simulink library "mbed_lib"  (Simulink 8.3)
settings: Solver=ode45  SolverMode=SingleTasking  StartTime=0.0  StopTime=10.0  RelTol=1e-3
settings Model: Creator=syoon  LastModifiedBy=axel

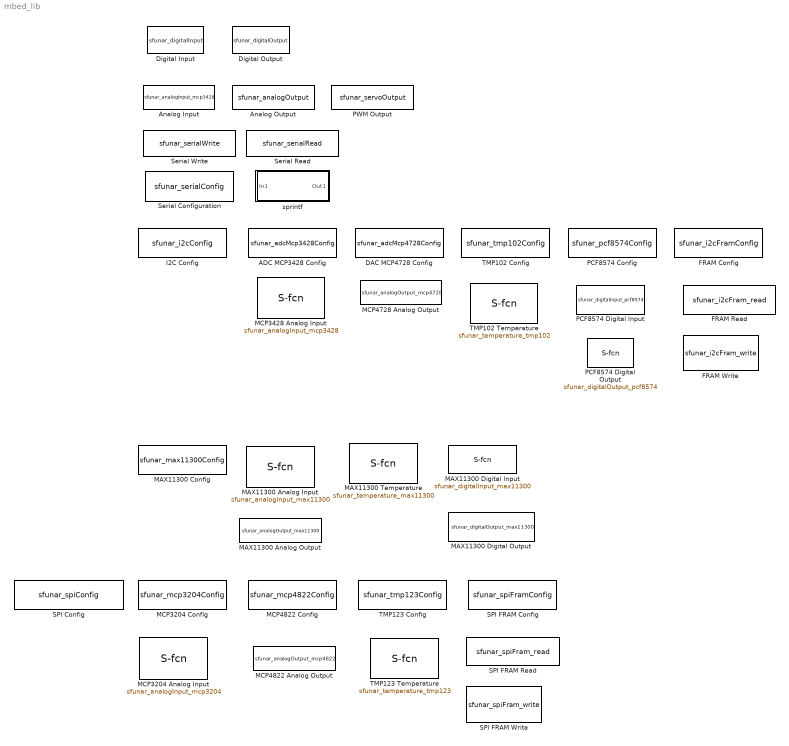
== system mbed_lib ==
  ADC MCP3428 Config : S-Function  Priority=1  AncestorBlock=mbed_lib/I2C Config  FunctionName=sfunar_adcMcp3428Config  Parameters=uint8(SParameter1)  EnableBusSupport=off  mask(MCP3428 Configuration){SParameter1=0}
      mask prompts: SParameter1 "Device Sub Address"
      mask help:
      | This blocks sets up the MCP3428 on the I2C board. You must have one of these blocks in any model that ues this device.
      |
      | The sub-address must match the pin configuration on the board. See the board documentation for details.
      mask Display: disp(['Sub-Address: ' num2str(SParameter1) ]);
  Analog Input : S-Function  FunctionName=sfunar_analogInput_mcp3428  Parameters=uint8(SParameter1), SampleTime  EnableBusSupport=off  mask(Arduino Analog Input){SParameter2=A, SParameter1=0, SampleTime=-1}
      mask prompts: SParameter2 "Port Name:"; SParameter1 "Pin Number (1-16):"; SampleTime "Sample time (-1 for inherited):"
      mask help:
      | Reads the analog voltage input from the specified pin on the Arduino board.
      |
      | The range of input on the pin is between 0 and 5 Volts corresponding to a block output of 0 to 1023.
      mask Help:
      | <p>This block calls the analogRead() function from the Arduino language library.
      | <p>For more information see: <a href="http://arduino.cc/en/Reference/AnalogRead">Arduino - AnalogRead</a>
      mask TypeOptions SParameter2: A | B | C | D | E | F
      mask Display:
      | plot([0:0.05:0.5],0.3*sin(4*pi*[0.5:0.05:1])+0.5)
      | port_label('output',1,['Pin ', SParameter2+64, '.', num2str(SParameter1)]);
  Analog Output : S-Function  FunctionName=sfunar_analogOutput  Parameters=uint8(SParameter1), SampleTime, uint8(SParameter2)  EnableBusSupport=off  mask(Arduino Analog Output){SParameter2=A, SampleTime=-1, SParameter1=0}
      mask prompts: SParameter2 "Port Name:"; SampleTime "Sample time (-1 for inherited):"; SParameter1 "Pin Number (1-16):"
      mask help:
      | Approximates an analog output on the specified pin on the Arduino board using a PWM signal with a frequency of ~490 Hz.
      |
      | The input to this block is an integer between 0 and 255 corresponding to 0 to 5V.
      mask Help:
      | <p>This block calls the analogWrite() function from the Arduino language library.
      | <p>For more information see: <a href="http://arduino.cc/en/Reference/AnalogWrite">Arduino - AnalogWrite</a>
      mask TypeOptions SParameter2: A | B | C | D | E | F
      mask Display:
      | plot([0.5:0.05:1],0.3*sin(4*pi*[0.5:0.05:1])+0.5)
      | port_label('input',1,['Pin ', SParameter2+64, '.', num2str(SParameter1)]);
  DAC MCP4728 Config : S-Function  Priority=1  FunctionName=sfunar_adcMcp4728Config  Parameters=uint8(SParameter1)  EnableBusSupport=off  mask(MCP4728 Configuration){SParameter1=0}
      mask prompts: SParameter1 "Device Sub Address"
      mask help:
      | This blocks sets up the MCP4728 on the I2C board. You must have one of these blocks in any model that ues this device.
      |
      | The sub-address must match the pin configuration on the board. See the board documentation for details.
      mask Display: disp(['Sub-Address: ' num2str(SParameter1) ]);
  Digital Input : S-Function  FunctionName=sfunar_digitalInput  Parameters=uint8(SParameter1), SampleTime, uint8(SParameter2), uint8(SParameter3)  EnableBusSupport=off  mask(Arduino Digital Input){SParameter2=A, SParameter1=0, SParameter3=INPUT, SampleTime=-1}
      mask prompts: SParameter2 "Port Name"; SParameter1 "Pin Number (1-16):"; SParameter3 "Input Mode"; SampleTime "Sample time (-1 for inherited):"
      mask help:
      | Reads the digital value from the specified pin on the Arduino board.
      |
      | It outputs 1 for high and 0 for low.
      mask Help:
      | <p>This block calls the digitalRead() function from the Arduino language library.
      | <p>For more information see: <a href="http://arduino.cc/en/Reference/DigitalRead">Arduino - DigitalRead</a>
      mask TypeOptions SParameter2: A | B | C | D | E | F
      mask TypeOptions SParameter3: INPUT | INPUT_PULLUP | INPUT_PULLDOWN
      mask Display:
      | plot([0 0.15 0.15 0.35 0.35 0.5],[0.3 0.3 0.7 0.7 0.3 0.3])
      | port_label('output',1,['Pin ', SParameter2+64, '.', num2str(SParameter1)]);
  Digital Output : S-Function  FunctionName=sfunar_digitalOutput  Parameters=uint8(SParameter1), SampleTime, uint8(SParameter2), uint8(SParameter3)  EnableBusSupport=off  mask(Arduino Digital Output){SParameter2=D, SParameter1=12, SParameter3=OUTPUT, SampleTime=-1}
      mask prompts: SParameter2 "Port Name:"; SParameter1 "Pin Number(1~16):"; SParameter3 "Output Mode"; SampleTime "Sample time (-1 for inherited):"
      mask help:
      | Sends the digital value to the specified port.pin on the Arduino board.
      | The pin can be configured as push-pull (pp) or open drain output (od).
      |
      | An input of 1 sets the pin high and 0 sets the pin low.
      mask Help:
      | <p>This block calls the digitalWrite() function from the Arduino language library.
      | <p>For init the pinmode function ist called
      | <p>For more information see: <a href="http://arduino.cc/en/Reference/DigitalWrite">Arduino - DigitalWrite</a>
      mask TypeOptions SParameter2: A | B | C | D | E | F
      mask TypeOptions SParameter3: OUTPUT | OUTPUT_OPENDRAIN
      mask Display:
      | plot([0.5 0.65 0.65 0.85 0.85 1],[0.3 0.3 0.7 0.7 0.3 0.3])
      | port_label('input',1,['Pin ', SParameter2+64, '.', num2str(SParameter1)]);
  FRAM Config : S-Function  Priority=1  FunctionName=sfunar_i2cFramConfig  EnableBusSupport=off  mask(I2C Fram Config){}
  FRAM Read : S-Function  FunctionName=sfunar_i2cFram_read  Parameters=uint8(SParameter1-1), SampleTime, boolean(errEn)  EnableBusSupport=off  mask(Fram Read){SampleTime=-1, SParameter1=on startup, errEn=on}
      mask prompts: SampleTime "Sample time (-1 for inherited):"; SParameter1 "Read condition"; errEn "Enable error output port"
      mask help: Reads one byte from the FRAM.
      mask TypeOptions SParameter1: on startup | on each step
      mask Display:
      | port_label('input', 1, 'Page Address');
      | port_label('input', 2, 'Word Address');
      | 
      | port_label('output',1,'Value');
      | if errEn
      | port_label('output',2,'Error');
      | end
  FRAM Write : S-Function  FunctionName=sfunar_i2cFram_write  Parameters=uint8(SParameter1-1), SampleTime, boolean(errEn)  EnableBusSupport=off  mask(FRAM Write){SampleTime=-1, SParameter1=on startup, errEn=on}
      mask prompts: SampleTime "Sample time (-1 for inherited):"; SParameter1 "Write condition"; errEn "Enable error output port"
      mask help: Writes one byte to the FRAM
      mask TypeOptions SParameter1: on startup | on each step
      mask Display:
      | port_label('input', 1, 'Page Address');
      | port_label('input', 2, 'Word Address');
      | port_label('input', 3, 'Data');
      | 
      | if errEn
      | port_label('output',1,'Error');
      | end
  I2C Config : S-Function  Priority=0  AncestorBlock=mbed_lib/Serial Configuration  FunctionName=sfunar_i2cConfig  Parameters=uint8(0), uint8(SParameter2), uint8(SParameter3), uint8(SParameter4), uint8(SParameter5), SParameter6  EnableBusSupport=off  mask(I2C Configuration){SParameter6=100000, SParameter2=B, SParameter3=9, SParameter4=B, SParameter5=8}
      mask prompts: SParameter6 "Bus frequency: [Hz]"; SParameter2 "Port Name (SDA)"; SParameter3 "Pin Number (1-16):"; SParameter4 "Port Name (SCL)"; SParameter5 "Pin Number (1-16):"
      mask help: This blocks sets up the I2C connection on the mbed board. You must have one of these blocks in any model that ues I2C blocks.
      mask TypeOptions SParameter2: A | B | C | D | E | F
      mask TypeOptions SParameter3: 0 | 1 | 2 | 3 | 4 | 5 | 6 | 7 | 8 | 9 | 10 | 11 | 12 | 13 | 14 | 15
      mask TypeOptions SParameter4: A | B | C | D | E | F
      mask TypeOptions SParameter5: 0 | 1 | 2 | 3 | 4 | 5 | 6 | 7 | 8 | 9 | 10 | 11 | 12 | 13 | 14 | 15
      mask Display:
      | disp(['SDA: ' SParameter2+64 '.' num2str(SParameter3-1) ', SCL: ' SParameter4+64, '.' num2str(SParameter5-1) ' \n']);
      | disp(['\nFrequency: ' num2str(SParameter6) ' HZ']);
  MAX11300 Analog Input : S-Function  FunctionName=sfunar_analogInput_max11300  Parameters=mode-1, SampleTime, posPin-1, negPin-1, power-1, range-1, ref-1, boolean(ErrorOutputEnable)  EnableBusSupport=off  mask(MAX11300 Analog Input){SampleTime=-1, mode=Single-Ended, posPin=1, negPin=1, power=1, range=0 to +10, ref=Internal (2.5 V), ErrorOutputEnable=on}
      mask prompts: SampleTime "Sample time (-1 for inherited):"; posPin "positive input pin"; negPin "negative input pin"; power "Average samples"; ref "Reference voltage"; ErrorOutputEnable "Enable error output"
      mask help: Reads the analog voltage input from the specified pin on the MAX11300.
      mask TypeOptions mode: Single-Ended | Differential
      mask TypeOptions posPin: 0 | 1 | 2 | 3 | 4 | 5 | 6 | 7 | 8 | 9 | 10 | 11 | 12 | 13 | 14 | 15 | 16 | 17 | 18 | 19
      mask TypeOptions negPin: 0 | 1 | 2 | 3 | 4 | 5 | 6 | 7 | 8 | 9 | 10 | 11 | 12 | 13 | 14 | 15 | 16 | 17 | 18 | 19
      mask TypeOptions power: 1 | 2 | 4 | 8 | 16 | 32 | 64 | 128
      mask TypeOptions range: Non selected | 0 to +10 | -5 to +5 | -10 to 0 | 0 to +2.5 | --- | 0 to +2.5 | ---
      mask TypeOptions ref: Internal (2.5 V) | External
      mask Display:
      | plot([0:0.01:0.25],0.3*sin(2*pi*[0:0.04:1])+0.5)
      | %disp(['Pin ', num2str(SParameter1-1)]);
      | port_label('output',1,'RAW');
      | port_label('output',2,'0-1');
      | if ErrorOutputEnable
      |     port_label('output',3,'Error');
      | end
  MAX11300 Analog Output : S-Function  FunctionName=sfunar_analogOutput_max11300  Parameters=pin-1, SampleTime, boolean(errEn), uint8(inputVariant-1), range-1  EnableBusSupport=off  mask(MAX11300 Analog Output){SampleTime=-1, pin=0, inputVariant=Uint16: left aligned (0x0YYY), range=0 to +10 V, errEn=on}
      mask prompts: SampleTime "Sample time (-1 for inherited):"; pin "Pin Number:"; inputVariant "Input data format"; errEn "Enable error output port"
      mask help:
      | Approximates an analog output on the specified pin on the MAX11300.
      |
      | Note: It can take up to 1 ms before the output voltage is updated on the pin.
      mask TypeOptions pin: 0 | 1 | 2 | 3 | 4 | 5 | 6 | 7 | 8 | 9 | 10 | 11 | 12 | 13 | 14 | 15 | 16 | 17 | 18 | 19
      mask TypeOptions inputVariant: Uint16: left aligned (0x0YYY) | Uint16: right aligned (0xYYY0) | Double: 0 ... 1
      mask TypeOptions range: Non selected | 0 to +10 V | -5 to +5  | -10 to 0  | -5 to +5 | --- | 0 to +10 | ---
      mask Display:
      | plot([0.5-.125:0.01:0.75-.125],0.3*sin(2*pi*[0:0.04:1])+0.5)
      | port_label('input',1,['Pin ', num2str(pin-1)]);
      | if errEn
      |     port_label('output',1,'Error');
      | end
  MAX11300 Config : S-Function  Priority=1  FunctionName=sfunar_max11300Config  Parameters=CS_PORT, CS_PIN, ADCCONV-1, DACREF-1  EnableBusSupport=off  mask(MAX11300 Configuration){CS_PORT=B, CS_PIN=6, ADCCONV=200 kSPS, DACREF=Internal (2.5 V)}
      mask prompts: CS_PORT "Chip Select: Port"; CS_PIN "Pin"; ADCCONV "ADC Conversion Rate"; DACREF "DAC Reference"
      mask help: This blocks sets up the MAX11300. You must have one of these blocks in any model that ues this device.
      mask TypeOptions CS_PORT: A | B | C | D | E | F
      mask TypeOptions CS_PIN: 0 | 1 | 2 | 3 | 4 | 5 | 6 | 7 | 8 | 9 | 10 | 11 | 12 | 13 | 14 | 15
      mask TypeOptions ADCCONV: 200 kSPS | 250 kSPS | 333 kSPS | 400 kSPS
      mask TypeOptions DACREF: External | Internal (2.5 V)
      mask Display: disp(['Chip Select: ' CS_PORT+64, '.' num2str(CS_PIN-1)]);
  MAX11300 Digital Input : S-Function  FunctionName=sfunar_digitalInput_max11300  Parameters=pin-1, SampleTime, boolean(errEn), thres  EnableBusSupport=off  mask(MAX11300 Digital Input){SampleTime=-1, pin=0, thres=1638, errEn=on}
      mask prompts: SampleTime "Sample time (-1 for inherited):"; pin "Pin Number:"; thres "Threshold:"; errEn "Enable error output port"
      mask help:
      | Reads the digital value from the specified pin of the MAX11300.
      |
      | Note: The external voltage is compared to an internal reference which can be
      | controlled by the threshold.
      | The threshold must be a number between 0 and 4095 (2^12-1) corresponding to a voltage of 0 to 5 V.
      mask TypeOptions pin: 0 | 1 | 2 | 3 | 4 | 5 | 6 | 7 | 8 | 9 | 10 | 11 | 12 | 13 | 14 | 15 | 16 | 17 | 18 | 19
      mask Display:
      | port_label('output',1,['Pin ', num2str(pin-1), ' > ', num2str(thres*5/(2^12-1)), ' V']);
      | if errEn
      | port_label('output',2,'Error');
      | end
  MAX11300 Digital Output : S-Function  FunctionName=sfunar_digitalOutput_max11300  Parameters=pin-1, SampleTime, boolean(errEn), level  EnableBusSupport=off  mask(MAX11300 digital output){SampleTime=-1, pin=0, level=2^12-1, errEn=on}
      mask prompts: SampleTime "Sample time (-1 for inherited):"; pin "Pin Number:"; level "Output level:"; errEn "Enable error output port"
      mask help:
      | Set an digital pin of the MAX11300.
      |
      | Note: The external voltage is set to an internal reference which can be
      | controlled by the level.
      | The level must be a number between 0 and 4095 (2^12-1) corresponding to a voltage of 0 to 5 V.
      mask TypeOptions pin: 0 | 1 | 2 | 3 | 4 | 5 | 6 | 7 | 8 | 9 | 10 | 11 | 12 | 13 | 14 | 15 | 16 | 17 | 18 | 19
      mask Display:
      | disp(['H-Level = ', num2str(level*5/(2^12-1)), ' V']);
      | port_label('input',1,['Pin ', num2str(pin-1)]);
      | if errEn
      | port_label('output',1,'Error');
      | end
  MAX11300 Temperature : S-Function  FunctionName=sfunar_temperature_max11300  Parameters=chan, SampleTime, boolean(errEn)  EnableBusSupport=off  mask(MAX11300 Temperature Input){SampleTime=-1, chan=Internal, errEn=on}
      mask prompts: SampleTime "Sample time (-1 for inherited):"; chan "Channel"; errEn "Enable error output port"
      mask help: Reads the last conversation result of the MAX11300.
      mask TypeOptions chan: Internal | External 1 | External 2
      mask Display:
      | disp(['Temperature\nChannel: ' int2str(chan-1)]);
      | port_label('output',1,'RAW');
      | port_label('output',2,'°C');
      | if errEn
      | port_label('output',3,'Error');
      | end
  MCP3204 Analog Input : S-Function  FunctionName=sfunar_analogInput_mcp3204  Parameters=mode-1, SampleTime, pin-1, boolean(ErrorOutputEnable)  EnableBusSupport=off  mask(MCP3204 Analog Input){SampleTime=-1, mode=Single-Ended, pin=1, ErrorOutputEnable=on}
      mask prompts: SampleTime "Sample time (-1 for inherited):"; ErrorOutputEnable "Enable error output"
      mask help: Reads the analog voltage input from the specified pin on the MCP3204.
      mask TypeOptions mode: Differential | Single-Ended
      mask TypeOptions pin: 0 | 1 | 2 | 3
      mask Display:
      | plot([0:0.01:0.25],0.3*sin(2*pi*[0:0.04:1])+0.5)
      | %disp(['Pin ', num2str(SParameter1-1)]);
      | port_label('output',1,'RAW');
      | port_label('output',2,'0-1');
      | if ErrorOutputEnable
      |     port_label('output',3,'Error');
      | end
  MCP3204 Config : S-Function  Priority=1  FunctionName=sfunar_mcp3204Config  Parameters=CS_PORT, CS_PIN  EnableBusSupport=off  mask(MCP3204 Configuration){CS_PORT=B, CS_PIN=6}
      mask prompts: CS_PORT "Chip Select: Port"; CS_PIN "Pin"
      mask help: This blocks sets up the MCP3204. You must have one of these blocks in any model that ues this device.
      mask TypeOptions CS_PORT: A | B | C | D | E | F
      mask TypeOptions CS_PIN: 0 | 1 | 2 | 3 | 4 | 5 | 6 | 7 | 8 | 9 | 10 | 11 | 12 | 13 | 14 | 15
      mask Display: disp(['Chip Select: ' CS_PORT+64, '.' num2str(CS_PIN-1)]);
  MCP3428 Analog Input : S-Function  AncestorBlock=mbed_lib/Analog Input  FunctionName=sfunar_analogInput_mcp3428  Parameters=uint8(SParameter1-1), SampleTime, uint8(SParameter2), uint8(SParameter3), boolean(ErrorOutputEnable)  EnableBusSupport=off  mask(MCP3428 Analog Input){SampleTime=-1, SParameter1=0, SParameter2=240 SPS (12 bit), SParameter3=1X, ErrorOutputEnable=on}
      mask prompts: SampleTime "Sample time (-1 for inherited):"; SParameter1 "Pin Number:"; SParameter2 "Sample-Rate"; SParameter3 "PGA-Gain"; ErrorOutputEnable "Enable error output port"
      mask help:
      | Reads the analog voltage input from the specified pin on the MCP3428.
      |
      | Warning: This block waits for a complete conversation during the execution step.
      | If the sample time is too small it will have an impact on the step time of the whole model!
      mask TypeOptions SParameter1: 0 | 1 | 2 | 3 | 4 | 5 | 6 | 7
      mask TypeOptions SParameter2: 240 SPS (12 bit) | 60 SPS (14 bit) | 15 SPS (16 bit)
      mask TypeOptions SParameter3: 1X | 2X | 4X | 8X
      mask Display:
      | plot([0:0.01:0.25],0.3*sin(2*pi*[0:0.04:1])+0.5)
      | disp(['Pin ', num2str(SParameter1-1)]);
      | port_label('output',1,'RAW');
      | port_label('output',2,'V');
      | port_label('output',3,'0-1');
      | if ErrorOutputEnable
      |     port_label('output',4,'Error');
      | end
  MCP4728 Analog Output : S-Function  AncestorBlock=mbed_lib/Analog Output  FunctionName=sfunar_analogOutput_mcp4728  Parameters=uint8(SParameter1-1), SampleTime, boolean(errEn), uint8(inputVariant-1), boolean(internalRef-1), boolean(gain2x-1)  EnableBusSupport=off  mask(MCP4728 Analog Output){SampleTime=-1, SParameter1=0, inputVariant=Uint16: right aligned (0x0YYY), internalRef=VDD (3.3 V), gain2x=1X, errEn=on}
      mask prompts: SampleTime "Sample time (-1 for inherited):"; SParameter1 "Pin Number:"; inputVariant "Input data format"; internalRef "Reference voltage"; gain2x "Gain"; errEn "Enable error output port"
      mask help: Approximates an analog output on the specified pin on the MCP4728.
      mask TypeOptions SParameter1: 0 | 1 | 2 | 3
      mask TypeOptions inputVariant: Uint16: right aligned (0x0YYY) | Uint16: left aligned (0xYYY0) | Double: Voltage in V | Double: 0 ... 1
      mask TypeOptions internalRef: VDD (3.3 V) | Internal (2.048 V)
      mask TypeOptions gain2x: 1X | 2X (only for internal VRef)
      mask Display:
      | plot([0.5-.125:0.01:0.75-.125],0.3*sin(2*pi*[0:0.04:1])+0.5)
      | port_label('input',1,['Pin ', num2str(SParameter1-1)]);
      | if errEn
      |     port_label('output',1,'Error');
      | end
  MCP4822 Analog Output : S-Function  FunctionName=sfunar_analogOutput_mcp4822  Parameters=pin-1, SampleTime, boolean(errEn), uint8(inputVariant-1), gain-1  EnableBusSupport=off  mask(MCP4822 Analog Output){SampleTime=-1, pin=0, inputVariant=Uint16: right aligned (0x0YYY), gain=1X, errEn=on}
      mask prompts: SampleTime "Sample time (-1 for inherited):"; pin "Pin Number:"; inputVariant "Input data format"; errEn "Enable error output port"
      mask help: Approximates an analog output on the specified pin on the MCP4822.
      mask TypeOptions pin: 0 | 1
      mask TypeOptions inputVariant: Uint16: right aligned (0x0YYY) | Uint16: left aligned (0xYYY0) | Double: 0 ... 1
      mask TypeOptions gain: 2X | 1X
      mask Display:
      | plot([0.5-.125:0.01:0.75-.125],0.3*sin(2*pi*[0:0.04:1])+0.5)
      | port_label('input',1,['Pin ', num2str(pin-1)]);
      | if errEn
      |     port_label('output',1,'Error');
      | end
  MCP4822 Config : S-Function  Priority=1  FunctionName=sfunar_mcp4822Config  Parameters=CS_PORT, CS_PIN  EnableBusSupport=off  mask(MCP4822 Configuration){CS_PORT=B, CS_PIN=6}
      mask prompts: CS_PORT "Chip Select: Port"; CS_PIN "Pin"
      mask help: This blocks sets up the MCP4822. You must have one of these blocks in any model that ues this device.
      mask TypeOptions CS_PORT: A | B | C | D | E | F
      mask TypeOptions CS_PIN: 0 | 1 | 2 | 3 | 4 | 5 | 6 | 7 | 8 | 9 | 10 | 11 | 12 | 13 | 14 | 15
      mask Display: disp(['Chip Select: ' CS_PORT+64, '.' num2str(CS_PIN-1)]);
  PCF8574 Config : S-Function  Priority=1  FunctionName=sfunar_pcf8574Config  Parameters=uint8(SParameter1)  EnableBusSupport=off  mask(PCF8574 Configuration){SParameter1=0}
      mask prompts: SParameter1 "Device Sub Address"
      mask help:
      | This blocks sets up the PCF8574 on the I2C board. You must have one of these blocks in any model that ues this device.
      |
      | The sub-address must match the pin configuration on the board. See the board documentation for details.
      mask Display: disp(['Sub-Address: ' num2str(SParameter1) ]);
  PCF8574 Digital Input : S-Function  FunctionName=sfunar_digitalInput_pcf8574  Parameters=uint8(SParameter1-1), SampleTime, boolean(errEn)  EnableBusSupport=off  mask(PCF8574 Digital Input){SampleTime=-1, SParameter1=0, errEn=on}
      mask prompts: SampleTime "Sample time (-1 for inherited):"; SParameter1 "Pin Number:"; errEn "Enable error output port"
      mask help:
      | Reads the digital value from the specified pin of the PCF8574.
      |
      | Note: The PCF8574 has an pull up current source on each pin.
      mask TypeOptions SParameter1: 0 | 1 | 2 | 3 | 4 | 5 | 6 | 7
      mask Display:
      | disp(['Pin ', num2str(SParameter1-1)]);
      | port_label('output',1,'Value');
      | if errEn
      | port_label('output',2,'Error');
      | end
  PCF8574 Digital Output : S-Function  FunctionName=sfunar_digitalOutput_pcf8574  Parameters=uint8(SParameter1-1), SampleTime, boolean(errEn)  EnableBusSupport=off  mask(PCF8574 digital output){SampleTime=-1, SParameter1=0, errEn=on}
      mask prompts: SampleTime "Sample time (-1 for inherited):"; SParameter1 "Pin Number:"; errEn "Enable error output port"
      mask help:
      | Set an digital pin of the PCF8574.
      |
      | Note: The PCF8574 has a high level output current of max. 300 µA but it can sink up to 25 mA on a low level output.
      mask TypeOptions SParameter1: 0 | 1 | 2 | 3 | 4 | 5 | 6 | 7
      mask Display:
      | port_label('input',1,['Pin ', num2str(SParameter1-1)]);
      | if errEn
      | port_label('output',1,'Error');
      | end
  PWM Output : S-Function  FunctionName=sfunar_servoOutput  Parameters=uint8(SParameter1), SampleTime  EnableBusSupport=off  mask(Arduino Analog Output){SParameter1=PA07 (TIM14_CH1), SampleTime=-1}
      mask prompts: SParameter1 "PWM Pin:"; SampleTime "Sample time (-1 for inherited):"
      mask help:
      | Approximates an analog output on the specified pin on the Arduino board using a PWM signal with a frequency of ~490 Hz.
      |
      | The input to this block is an integer between 0 and 255 corresponding to 0 to 5V.
      mask Help:
      | <p>This block calls the analogWrite() function from the Arduino language library.
      | <p>For more information see: <a href="http://arduino.cc/en/Reference/AnalogWrite">Arduino - AnalogWrite</a>
      mask TypeOptions SParameter1: PA07 (TIM14_CH1) | PA08 (TIM1_CH1) | PB00 (TIM3_CH3) | PB01 (TIM3_CH4) | PB04 (TIM3_CH1) | PB05 (TIM3_CH2) | PC06 (TIM8_CH1) | PC07 (TIM8_CH2) | PC08 (TIM8_CH3) | PC09 (TIM8_CH4) | PD12 (TIM4_CH1) | PD13 (TIM4_CH2) | PD14 (TIM4_CH3) | PD15 (TIM4_CH4) | PE13 (TIM1_CH3) | PE14 (TIM1_CH4)
      mask Display:
      | plot([0.5 0.65 0.65 0.85 ],[0.3 0.3 0.7 0.7 ])
      | plot([0.8 0.8],[0.7 0.3])
      | plot([0.825 0.825],[0.7 0.3])
      | plot([0.85 0.85],[0.7 0.3])
      | plot([0.8 1],[0.3 0.3])
      | p={'PA07';'PA08';'PB00';'PB01';'PB04';'PB05';'PC06';'PC07';'PC08';'PC09';'PD12';'PD13';'PD14';'PD15';'PE13';'PE14'};
      | port_label('input',1,[p{SParameter1}]);
  SPI Config : S-Function  Priority=0  FunctionName=sfunar_spiConfig  Parameters=uint8(0), uint8(SParameter2), uint8(SParameter3), uint8(SParameter4), uint8(SParameter5), SParameter6, uint8(SCK_PORT), uint8(SCK_PIN)  EnableBusSupport=off  mask(SPI Configuration){SParameter6=100000, SParameter2=A, SParameter3=7, SParameter4=A, SParameter5=6, SCK_PORT=A, SCK_PIN=5}
      mask prompts: SParameter6 "Bus frequency: [Hz]"; SParameter2 "MOSI: Port"; SParameter3 "Pin"; SParameter4 "MISO: Port"; SParameter5 "Pin"; SCK_PORT "SCK: Port"; SCK_PIN "Pin"
      mask help: This blocks sets up the SPI connection on the mbed board. You must have one of these blocks in any model that ues SPI blocks.
      mask TypeOptions SParameter2: A | B | C | D | E | F
      mask TypeOptions SParameter3: 0 | 1 | 2 | 3 | 4 | 5 | 6 | 7 | 8 | 9 | 10 | 11 | 12 | 13 | 14 | 15
      mask TypeOptions SParameter4: A | B | C | D | E | F
      mask TypeOptions SParameter5: 0 | 1 | 2 | 3 | 4 | 5 | 6 | 7 | 8 | 9 | 10 | 11 | 12 | 13 | 14 | 15
      mask TypeOptions SCK_PORT: A | B | C | D | E | F
      mask TypeOptions SCK_PIN: 0 | 1 | 2 | 3 | 4 | 5 | 6 | 7 | 8 | 9 | 10 | 11 | 12 | 13 | 14 | 15
      mask Display:
      | disp(['MOSI: ' SParameter2+64 '.' num2str(SParameter3-1) ', MISO: ' SParameter4+64, '.' num2str(SParameter5-1)  ', SCK: ' SCK_PORT+64, '.' num2str(SCK_PIN-1) ' \n']);
      | disp(['\nFrequency: ' num2str(SParameter6) ' HZ']);
  SPI FRAM Config : S-Function  Priority=1  FunctionName=sfunar_spiFramConfig  Parameters=CS_PORT, CS_PIN  EnableBusSupport=off  mask(SPI FRAM Configuration){CS_PORT=B, CS_PIN=6}
      mask prompts: CS_PORT "Chip Select: Port"; CS_PIN "Pin"
      mask help: This blocks sets up the FRAM. You must have one of these blocks in any model that ues this device.
      mask TypeOptions CS_PORT: A | B | C | D | E | F
      mask TypeOptions CS_PIN: 0 | 1 | 2 | 3 | 4 | 5 | 6 | 7 | 8 | 9 | 10 | 11 | 12 | 13 | 14 | 15
      mask Display: disp(['Chip Select: ' CS_PORT+64, '.' num2str(CS_PIN-1)]);
  SPI FRAM Read : S-Function  FunctionName=sfunar_spiFram_read  Parameters=uint8(SParameter1-1), SampleTime, boolean(errEn)  EnableBusSupport=off  mask(FRAM Read){SampleTime=-1, SParameter1=on startup, errEn=on}
      mask prompts: SampleTime "Sample time (-1 for inherited):"; SParameter1 "Read condition"; errEn "Enable error output port"
      mask help: Reads one byte from the FRAM
      mask TypeOptions SParameter1: on startup | on each step
      mask Display:
      | port_label('input', 1, 'Page Address');
      | port_label('input', 2, 'Word Address');
      | 
      | port_label('output',1,'Value');
      | if errEn
      | port_label('output',2,'Error');
      | end
  SPI FRAM Write : S-Function  FunctionName=sfunar_spiFram_write  Parameters=uint8(SParameter1-1), SampleTime, boolean(errEn)  EnableBusSupport=off  mask(FRAM write){SampleTime=-1, SParameter1=on startup, errEn=on}
      mask prompts: SampleTime "Sample time (-1 for inherited):"; SParameter1 "Write condition"; errEn "Enable error output port"
      mask help: Writes one byte to the FRAM
      mask TypeOptions SParameter1: on startup | on each step
      mask Display:
      | port_label('input', 1, 'Page Address');
      | port_label('input', 2, 'Word Address');
      | port_label('input', 3, 'Data');
      | 
      | if errEn
      | port_label('output',1,'Error');
      | end
  Serial Configuration : S-Function  FunctionName=sfunar_serialConfig  Parameters=uint8(SParameter1), uint8(SParameter2), uint8(SParameter3), uint8(SParameter4), uint8(SParameter5), SParameter6  EnableBusSupport=off  mask(Arduino Serial Configuration){SParameter1=1, SParameter6=9600, SParameter2=A, SParameter3=3, SParameter4=A, SParameter5=4}
      mask prompts: SParameter1 "Serial Port"; SParameter6 "Baud Rate:"; SParameter2 "Port Name (TX)"; SParameter3 "Pin Number (1-16):"; SParameter4 "Port Name (RX)"; SParameter5 "Pin Number (1-16):"
      mask help:
      | This blocks sets up the serial connection on the Arduino board. You must have one of these blocks in any model that ues the Serial Send or Serial Read blocks.
      |
      | Set the baud rate to match the device that you are communicating with. Standard rates include:300, 1200, 2400, 4800, 9600, 14400, 19200, 28800, 38400, 57600, or 115200.
      mask Help:
      | <p>This block calls the Serial.begin() function from the Arduino language library.
      | <p>For more information see: <a href="http://arduino.cc/en/Serial/Begin">Arduino - Serial/Begin</a>
      mask TypeOptions SParameter1: 1 | 2 | 3 | 4 | 5
      mask TypeOptions SParameter2: A | B | C | D | E | F
      mask TypeOptions SParameter3: 0 | 1 | 2 | 3 | 4 | 5 | 6 | 7 | 8 | 9 | 10 | 11 | 12 | 13 | 14 | 15
      mask TypeOptions SParameter4: A | B | C | D | E | F
      mask TypeOptions SParameter5: 0 | 1 | 2 | 3 | 4 | 5 | 6 | 7 | 8 | 9 | 10 | 11 | 12 | 13 | 14 | 15
      mask Display:
      | disp(['Serial Config ' num2str(SParameter1) '\n\n']);
      | disp(['TX ' SParameter2+64 '.' num2str(SParameter3-1) ', RX ' SParameter4+64, '.' num2str(SParameter5-1)]);
  Serial Read : S-Function  FunctionName=sfunar_serialRead  Parameters=SampleTime, uint8(SParameter1)  EnableBusSupport=off  mask(Arduino Serial Read){SParameter1=USB, SampleTime=-1}
      mask prompts: SParameter1 "Serial Port"; SampleTime "Sample time (-1 for inherited):"
      mask help:
      | Reads one byte from the serial interface on the Arduino board.
      |
      | Outputs -1 if no data is available to be read.
      mask Help:
      | <p>This block calls the Serial.read() function from the Arduino language library.
      | <p>For more information see: <a href="http://arduino.cc/en/Serial/Read">Arduino - Serial/Read</a>
      mask TypeOptions SParameter1: USB | UART1(A2,A3) | USART3(D8,D9)
      mask Display:
      | p={'USB'; 'UART1'; 'USART3'};
      | disp(['Serial Read ' p{SParameter1}])
  Serial Write : S-Function  FunctionName=sfunar_serialWrite  Parameters=SampleTime, uint8(SParameter1)  EnableBusSupport=off  mask(Arduino Serial Write){SParameter1=USB, SampleTime=-1}
      mask prompts: SParameter1 "Serial Port"; SampleTime "Sample time (-1 for inherited):"
      mask help:
      | Writes a vector of bytes to the serial port on the Arduino board.
      |
      | Outputs -1 if no data is available to be read.
      mask Help:
      | <p>This block calls the Serial.write() function from the Arduino language library.
      | <p>For more information see: <a href="http://arduino.cc/en/Serial/Write">Arduino - Serial/Write</a>
      mask TypeOptions SParameter1: USB | UART1(A2,A3) | USART3(D8,D9)
      mask Display:
      | p={'USB'; 'UART1'; 'USART3'};
      | disp(['Serial Write ' p{SParameter1}])
  TMP102 Config : S-Function  Priority=1  FunctionName=sfunar_tmp102Config  Parameters=uint8(SParameter1), uint8(SParameter2)  EnableBusSupport=off  mask(TMP102 Configuration){SParameter1=0, SParameter2=4 Hz}
      mask prompts: SParameter1 "Device Sub Address"; SParameter2 "Samplerate"
      mask help:
      | This blocks sets up the TMP102 on the I2C board. You must have one of these blocks in any model that ues this device.
      |
      | The sub-address must match the pin configuration on the board. See the board documentation for details.
      mask TypeOptions SParameter2: 0.25 Hz | 1 Hz | 4 Hz | 8 Hz
      mask Display: disp(['Sub-Address: ' num2str(SParameter1) ]);
  TMP102 Temperature : S-Function  FunctionName=sfunar_temperature_tmp102  Parameters=uint8(0), SampleTime, boolean(errEn)  EnableBusSupport=off  mask(TMP102 Temperature Input){SampleTime=-1, errEn=on}
      mask prompts: SampleTime "Sample time (-1 for inherited):"; errEn "Enable error output port"
      mask help:
      | Reads the last conversation result of the TMP102.
      |
      | Warning: The TMP102 needs at least 26 ms for one conversation.
      | If the sample time for this block is faster than this time the sensor may not produce valid values.
      mask Display:
      | disp(['Temperature']);
      | port_label('output',1,'RAW');
      | port_label('output',2,'°C');
      | if errEn
      | port_label('output',3,'Error');
      | end
  TMP123 Config : S-Function  Priority=1  FunctionName=sfunar_tmp123Config  Parameters=CS_PORT, CS_PIN  EnableBusSupport=off  mask(TMP123 Configuration){CS_PORT=B, CS_PIN=6}
      mask prompts: CS_PORT "Chip Select: Port"; CS_PIN "Pin"
      mask help: This blocks sets up the TMP123. You must have one of these blocks in any model that ues this device.
      mask TypeOptions CS_PORT: A | B | C | D | E | F
      mask TypeOptions CS_PIN: 0 | 1 | 2 | 3 | 4 | 5 | 6 | 7 | 8 | 9 | 10 | 11 | 12 | 13 | 14 | 15
      mask Display: disp(['Chip Select: ' CS_PORT+64, '.' num2str(CS_PIN-1)]);
  TMP123 Temperature : S-Function  FunctionName=sfunar_temperature_tmp123  Parameters=uint8(0), SampleTime, boolean(errEn)  EnableBusSupport=off  mask(TMP123 Temperature Input){SampleTime=-1, errEn=on}
      mask prompts: SampleTime "Sample time (-1 for inherited):"; errEn "Enable error output port"
      mask help:
      | Reads the last conversation result of the TMP123.
      |
      | Warning: The TMP123 needs 320 ms max for one conversation.
      | If the sample time for this block is faster than this time the sensor may not produce valid values.
      mask Display:
      | disp(['Temperature']);
      | port_label('output',1,'RAW');
      | port_label('output',2,'°C');
      | if errEn
      | port_label('output',3,'Error');
      | end
  sprintf : Subsystem  mask{format=%f}
      mask TypeOptions format: %f | %d
      mask Display:
      | p={'%f'; '%d'};
      | disp(['sprintf: ' p{format}])

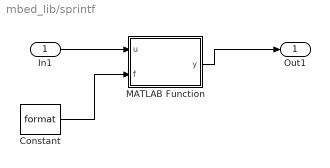
== system mbed_lib/sprintf ==
  In1 : Inport
  Constant : Constant  Value=format
  MATLAB Function : MATLAB Function  TreatAsAtomicUnit=on
  Out1 : Outport
  wires:
  In1/1 -> MATLAB Function/1(u)
  MATLAB Function/1(y) -> Out1/1
  Constant/1 -> MATLAB Function/2(f)

== matlab function sprintf/MATLAB Function ==
  data: u input double; y output double; f input double
function y = fcn(u,f)
buffer = char(zeros(1,15));
% geht mit 2012b noch nicht aber mit 2014a oder 2013: coder.cinclude('stdio.h');
coder.ceval('#ifdef _WIN32 //');
  if f == 1
    coder.ceval('_snprintf', coder.ref(buffer(int32(1))),int32(size(buffer,2)), ['%f' char(13) char(10) 0], u);
  elseif f==2
    coder.ceval('_snprintf', coder.ref(buffer(int32(1))),int32(size(buffer,2)), ['%d' char(13) char(10) 0], u);
  end
coder.ceval('#else //');
  if f == 1
    coder.ceval('snprintf', coder.ref(buffer(int32(1))),int32(size(buffer,2)), ['%f' char(13) char(10) 0], u);
  elseif f==2
    coder.ceval('snprintf', coder.ref(buffer(int32(1))),int32(size(buffer,2)), ['%d' char(13) char(10) 0], u);
  end
coder.ceval('#endif //');
y = uint8(buffer);
